simulink model "Lab-1"  (R2023a)
settings: Solver=VariableStepAuto  StartTime=0.0  StopTime=0.25  RelTol=1e-3
settings Model: Creator=ПК  LastModifiedBy=ПК

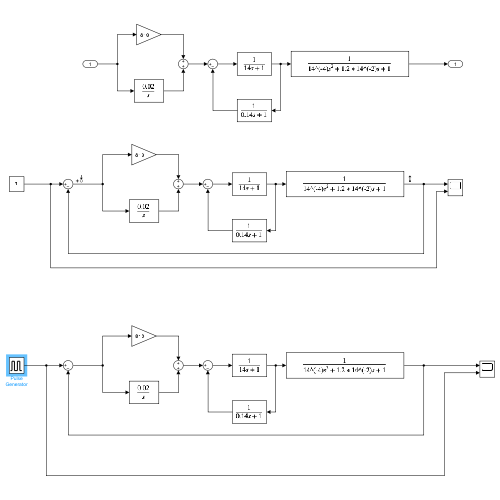
[thumbnail: Simulink's stored preview of the top-level diagram]
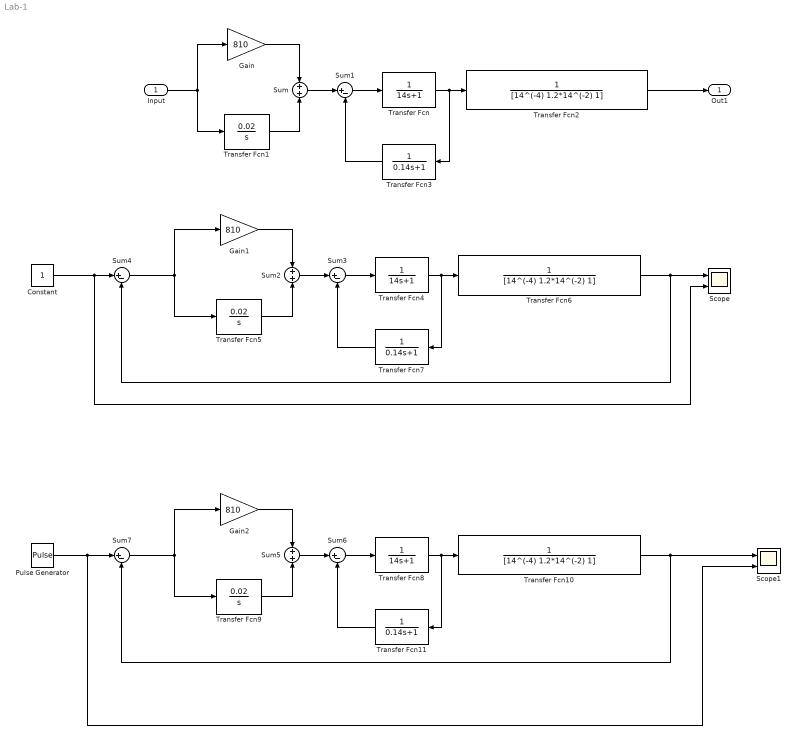
== system Lab-1 ==
  Input : Inport
  Constant : Constant
  Gain : Gain  Gain=810
  Gain1 : Gain  Gain=810
  Gain2 : Gain  Gain=810
  Pulse Generator : DiscretePulseGenerator  PulseType=Time based  Period=10  PulseWidth=0.01
  Scope : Scope  NumInputPorts=2
  Scope1 : Scope  NumInputPorts=2
  Sum : Sum
  Sum{1,3..4,6..7} (5 alike) : Sum  Inputs=|+-
  Sum2 : Sum
  Sum5 : Sum
  Transfer Fcn : TransferFcn  Denominator=[14 1]
  Transfer Fcn1 : TransferFcn  Numerator=0.02  Denominator=[1 0]
  Transfer Fcn10 : TransferFcn  Denominator=[14^(-4) 1.2*14^(-2) 1]
  Transfer Fcn11 : TransferFcn  Denominator=[0.14 1]
  Transfer Fcn2 : TransferFcn  Denominator=[14^(-4) 1.2*14^(-2) 1]
  Transfer Fcn3 : TransferFcn  Denominator=[0.14 1]
  Transfer Fcn4 : TransferFcn  Denominator=[14 1]
  Transfer Fcn5 : TransferFcn  Numerator=0.02  Denominator=[1 0]
  Transfer Fcn6 : TransferFcn  Denominator=[14^(-4) 1.2*14^(-2) 1]
  Transfer Fcn7 : TransferFcn  Denominator=[0.14 1]
  Transfer Fcn8 : TransferFcn  Denominator=[14 1]
  Transfer Fcn9 : TransferFcn  Numerator=0.02  Denominator=[1 0]
  Out1 : Outport
  wires:
  Gain/1 -> Sum/1
  Sum/1 -> Sum1/1
  Sum1/1 -> Transfer Fcn/1
  Transfer Fcn1/1 -> Sum/2
  Transfer Fcn/1 -> Transfer Fcn3/1, Transfer Fcn2/1
  Transfer Fcn3/1 -> Sum1/2
  Input/1 -> Transfer Fcn1/1, Gain/1
  Transfer Fcn2/1 -> Out1/1
  Transfer Fcn6/1 -> Scope/1, Sum4/2
  Transfer Fcn4/1 -> Transfer Fcn7/1, Transfer Fcn6/1
  Transfer Fcn7/1 -> Sum3/2
  Gain1/1 -> Sum2/1
  Sum3/1 -> Transfer Fcn4/1
  Sum2/1 -> Sum3/1
  Transfer Fcn5/1 -> Sum2/2
  Sum4/1 -> Transfer Fcn5/1, Gain1/1
  Constant/1 -> Scope/2, Sum4/1
  Pulse Generator/1 -> Scope1/2, Sum7/1
  Transfer Fcn8/1 -> Transfer Fcn11/1, Transfer Fcn10/1
  Sum5/1 -> Sum6/1
  Gain2/1 -> Sum5/1
  Transfer Fcn11/1 -> Sum6/2
  Transfer Fcn9/1 -> Sum5/2
  Sum6/1 -> Transfer Fcn8/1
  Transfer Fcn10/1 -> Scope1/1, Sum7/2
  Sum7/1 -> Transfer Fcn9/1, Gain2/1
